simulink model "fuzzy_controller_7_trimf"  (Simulink 7.2)
settings: Solver=ode45  StartTime=0.0  StopTime=10.0  RelTol=1e-3
values from neighbouring files (symbols this model uses):
  fi_1_a = -0.786    [fuzzy_controller_3_trimf_params.m]    (also in fuzzy_controller_5_gbell_params.m = 0.1768; fuzzy_controller_5_trimf_optimal_params.m; fuzzy_controller_5_trimf_params.m; fuzzy_controller_7_trimf_params.m)
  fi_1_b = -0.786    [fuzzy_controller_3_trimf_params.m]    (also in fuzzy_controller_5_gbell_params.m = 3.278; fuzzy_controller_5_trimf_optimal_params.m; fuzzy_controller_5_trimf_params.m; fuzzy_controller_7_trimf_params.m)
  fi_1_c = 0    [fuzzy_controller_3_trimf_params.m]    (also in fuzzy_controller_5_gbell_params.m = -0.7664; fuzzy_controller_5_trimf_optimal_params.m = -0.1; fuzzy_controller_5_trimf_params.m = -0.393; fuzzy_controller_7_trimf_params.m = -0.523)
  fi_2_a = -0.786    [fuzzy_controller_3_trimf_params.m]    (also in fuzzy_controller_5_gbell_params.m = 0.1965; fuzzy_controller_5_trimf_optimal_params.m = -0.1; fuzzy_controller_5_trimf_params.m; fuzzy_controller_7_trimf_params.m)
  fi_2_b = 0    [fuzzy_controller_3_trimf_params.m]    (also in fuzzy_controller_5_gbell_params.m = 3.278; fuzzy_controller_5_trimf_optimal_params.m = -0.05; fuzzy_controller_5_trimf_params.m = -0.393; fuzzy_controller_7_trimf_params.m = -0.5238)
  fi_2_c = 0.786    [fuzzy_controller_3_trimf_params.m]    (also in fuzzy_controller_5_gbell_params.m = -0.393; fuzzy_controller_5_trimf_optimal_params.m = 0; fuzzy_controller_5_trimf_params.m = 0; fuzzy_controller_7_trimf_params.m = -0.262)
  fi_3_a = 0    [fuzzy_controller_3_trimf_params.m]    (also in fuzzy_controller_5_gbell_params.m = 0.1965; fuzzy_controller_5_trimf_optimal_params.m = -0.05; fuzzy_controller_5_trimf_params.m = -0.393; fuzzy_controller_7_trimf_params.m = -0.523)
  fi_3_b = 0.786    [fuzzy_controller_3_trimf_params.m]    (also in fuzzy_controller_5_gbell_params.m = 3.278; fuzzy_controller_5_trimf_optimal_params.m = 0; fuzzy_controller_5_trimf_params.m = 0; fuzzy_controller_7_trimf_params.m = -0.262)
  fi_3_c = 0.786    [fuzzy_controller_3_trimf_params.m]    (also in fuzzy_controller_5_gbell_params.m = 0; fuzzy_controller_5_trimf_optimal_params.m = 0.05; fuzzy_controller_5_trimf_params.m = 0.393; fuzzy_controller_7_trimf_params.m = 0)
  fi_4_a = 0.1965    [fuzzy_controller_5_gbell_params.m]    (also in fuzzy_controller_5_trimf_optimal_params.m = 0; fuzzy_controller_5_trimf_params.m = 0; fuzzy_controller_7_trimf_params.m = -0.262)
  fi_4_b = 3.278    [fuzzy_controller_5_gbell_params.m]    (also in fuzzy_controller_5_trimf_optimal_params.m = 0.05; fuzzy_controller_5_trimf_params.m = 0.393; fuzzy_controller_7_trimf_params.m = 0)
  fi_4_c = 0.393    [fuzzy_controller_5_gbell_params.m]    (also in fuzzy_controller_5_trimf_optimal_params.m = 0.1; fuzzy_controller_5_trimf_params.m = 0.786; fuzzy_controller_7_trimf_params.m = 0.262)
  fi_5_a = 0.1768    [fuzzy_controller_5_gbell_params.m]    (also in fuzzy_controller_5_trimf_optimal_params.m = 0.05; fuzzy_controller_5_trimf_params.m = 0.393; fuzzy_controller_7_trimf_params.m = 0)
  fi_5_b = 3.278    [fuzzy_controller_5_gbell_params.m]    (also in fuzzy_controller_5_trimf_optimal_params.m = 0.1; fuzzy_controller_5_trimf_params.m = 0.786; fuzzy_controller_7_trimf_params.m = 0.262)
  fi_5_c = 0.7664    [fuzzy_controller_5_gbell_params.m]    (also in fuzzy_controller_5_trimf_optimal_params.m = 0.786; fuzzy_controller_5_trimf_params.m = 0.786; fuzzy_controller_7_trimf_params.m = 0.523)
  fi_6_a = 0.262    [fuzzy_controller_7_trimf_params.m]
  fi_6_b = 0.523    [fuzzy_controller_7_trimf_params.m]
  fi_6_c = 0.786    [fuzzy_controller_7_trimf_params.m]
  fi_7_a = 0.523    [fuzzy_controller_7_trimf_params.m]
  fi_7_b = 0.786    [fuzzy_controller_7_trimf_params.m]
  fi_7_c = 0.786    [fuzzy_controller_7_trimf_params.m]
  FORCE_1_a = -150    [fuzzy_controller_3_trimf_params.m]    (also in fuzzy_controller_5_trimf_optimal_params.m; fuzzy_controller_5_trimf_params.m; fuzzy_controller_7_trimf_params.m)
  FORCE_1_b = -150    [fuzzy_controller_3_trimf_params.m]    (also in fuzzy_controller_5_trimf_optimal_params.m; fuzzy_controller_5_trimf_params.m; fuzzy_controller_7_trimf_params.m)
  FORCE_1_c = 0    [fuzzy_controller_3_trimf_params.m]    (also in fuzzy_controller_5_trimf_optimal_params.m = -75; fuzzy_controller_5_trimf_params.m = -75; fuzzy_controller_7_trimf_params.m = -100)
  FORCE_2_a = -150    [fuzzy_controller_3_trimf_params.m]    (also in fuzzy_controller_5_trimf_optimal_params.m; fuzzy_controller_5_trimf_params.m; fuzzy_controller_7_trimf_params.m)
  FORCE_2_b = 0    [fuzzy_controller_3_trimf_params.m]    (also in fuzzy_controller_5_trimf_optimal_params.m = -75; fuzzy_controller_5_trimf_params.m = -75; fuzzy_controller_7_trimf_params.m = -100)
  FORCE_2_c = 150    [fuzzy_controller_3_trimf_params.m]    (also in fuzzy_controller_5_trimf_optimal_params.m = 0; fuzzy_controller_5_trimf_params.m = 0; fuzzy_controller_7_trimf_params.m = -50)
  FORCE_3_a = 0    [fuzzy_controller_3_trimf_params.m]    (also in fuzzy_controller_5_trimf_optimal_params.m = -75; fuzzy_controller_5_trimf_params.m = -75; fuzzy_controller_7_trimf_params.m = -100)
  FORCE_3_b = 150    [fuzzy_controller_3_trimf_params.m]    (also in fuzzy_controller_5_trimf_optimal_params.m = 0; fuzzy_controller_5_trimf_params.m = 0; fuzzy_controller_7_trimf_params.m = -50)
  FORCE_3_c = 150    [fuzzy_controller_3_trimf_params.m]    (also in fuzzy_controller_5_trimf_optimal_params.m = 75; fuzzy_controller_5_trimf_params.m = 75; fuzzy_controller_7_trimf_params.m = 0)
  FORCE_4_a = 0    [fuzzy_controller_5_trimf_optimal_params.m]    (also in fuzzy_controller_5_trimf_params.m; fuzzy_controller_7_trimf_params.m = -50)
  FORCE_4_b = 75    [fuzzy_controller_5_trimf_optimal_params.m]    (also in fuzzy_controller_5_trimf_params.m; fuzzy_controller_7_trimf_params.m = 0)
  FORCE_4_c = 150    [fuzzy_controller_5_trimf_optimal_params.m]    (also in fuzzy_controller_5_trimf_params.m; fuzzy_controller_7_trimf_params.m = 50)
  FORCE_5_a = 75    [fuzzy_controller_5_trimf_optimal_params.m]    (also in fuzzy_controller_5_trimf_params.m; fuzzy_controller_7_trimf_params.m = 0)
  FORCE_5_b = 150    [fuzzy_controller_5_trimf_optimal_params.m]    (also in fuzzy_controller_5_trimf_params.m; fuzzy_controller_7_trimf_params.m = 50)
  FORCE_5_c = 150    [fuzzy_controller_5_trimf_optimal_params.m]    (also in fuzzy_controller_5_trimf_params.m; fuzzy_controller_7_trimf_params.m = 100)
  FORCE_6_a = 50    [fuzzy_controller_7_trimf_params.m]
  FORCE_6_b = 100    [fuzzy_controller_7_trimf_params.m]
  FORCE_6_c = 150    [fuzzy_controller_7_trimf_params.m]
  FORCE_7_a = 100    [fuzzy_controller_7_trimf_params.m]
  FORCE_7_b = 150    [fuzzy_controller_7_trimf_params.m]
  FORCE_7_c = 150    [fuzzy_controller_7_trimf_params.m]
  FORCE_Range_1 = -150    [fuzzy_controller_3_trimf_params.m]    (also in fuzzy_controller_5_gauss_params.m; fuzzy_controller_5_gbell_params.m; fuzzy_controller_5_trimf_optimal_params.m; fuzzy_controller_5_trimf_params.m)
  FORCE_Range_2 = 150    [fuzzy_controller_3_trimf_params.m]    (also in fuzzy_controller_5_gauss_params.m; fuzzy_controller_5_gbell_params.m; fuzzy_controller_5_trimf_optimal_params.m; fuzzy_controller_5_trimf_params.m)
  omega_1_a = -1.57    [fuzzy_controller_3_trimf_params.m]    (also in fuzzy_controller_5_gbell_params.m = 0.3532; fuzzy_controller_5_trimf_optimal_params.m; fuzzy_controller_5_trimf_params.m; fuzzy_controller_7_trimf_params.m)
  omega_1_b = -1.57    [fuzzy_controller_3_trimf_params.m]    (also in fuzzy_controller_5_gbell_params.m = 3.278; fuzzy_controller_5_trimf_optimal_params.m; fuzzy_controller_5_trimf_params.m; fuzzy_controller_7_trimf_params.m)
  omega_1_c = 0    [fuzzy_controller_3_trimf_params.m]    (also in fuzzy_controller_5_gbell_params.m = -1.531; fuzzy_controller_5_trimf_optimal_params.m = -0.86; fuzzy_controller_5_trimf_params.m = -0.785; fuzzy_controller_7_trimf_params.m = -1.047)
  omega_2_a = -1.57    [fuzzy_controller_3_trimf_params.m]    (also in fuzzy_controller_5_gbell_params.m = 0.3925; fuzzy_controller_5_trimf_optimal_params.m = -0.86; fuzzy_controller_5_trimf_params.m; fuzzy_controller_7_trimf_params.m)
  omega_2_b = 0    [fuzzy_controller_3_trimf_params.m]    (also in fuzzy_controller_5_gbell_params.m = 3.278; fuzzy_controller_5_trimf_optimal_params.m = -0.43; fuzzy_controller_5_trimf_params.m = -0.785; fuzzy_controller_7_trimf_params.m = -1.047)
  omega_2_c = 1.57    [fuzzy_controller_3_trimf_params.m]    (also in fuzzy_controller_5_gbell_params.m = -0.785; fuzzy_controller_5_trimf_optimal_params.m = 0; fuzzy_controller_5_trimf_params.m = 0; fuzzy_controller_7_trimf_params.m = -0.523)
  omega_3_a = 0    [fuzzy_controller_3_trimf_params.m]    (also in fuzzy_controller_5_gbell_params.m = 0.3925; fuzzy_controller_5_trimf_optimal_params.m = -0.43; fuzzy_controller_5_trimf_params.m = -0.785; fuzzy_controller_7_trimf_params.m = -1.047)
  omega_3_b = 1.57    [fuzzy_controller_3_trimf_params.m]    (also in fuzzy_controller_5_gbell_params.m = 3.278; fuzzy_controller_5_trimf_optimal_params.m = 0; fuzzy_controller_5_trimf_params.m = 0; fuzzy_controller_7_trimf_params.m = -0.523)
  omega_3_c = 1.57    [fuzzy_controller_3_trimf_params.m]    (also in fuzzy_controller_5_gbell_params.m = 0; fuzzy_controller_5_trimf_optimal_params.m = 0.43; fuzzy_controller_5_trimf_params.m = 0.785; fuzzy_controller_7_trimf_params.m = 0)
  omega_4_a = 0.3925    [fuzzy_controller_5_gbell_params.m]    (also in fuzzy_controller_5_trimf_optimal_params.m = 0; fuzzy_controller_5_trimf_params.m = 0; fuzzy_controller_7_trimf_params.m = -0.523)
  omega_4_b = 3.278    [fuzzy_controller_5_gbell_params.m]    (also in fuzzy_controller_5_trimf_optimal_params.m = 0.43; fuzzy_controller_5_trimf_params.m = 0.785; fuzzy_controller_7_trimf_params.m = 0)
  omega_4_c = 0.785    [fuzzy_controller_5_gbell_params.m]    (also in fuzzy_controller_5_trimf_optimal_params.m = 0.86; fuzzy_controller_5_trimf_params.m = 1.57; fuzzy_controller_7_trimf_params.m = 0.523)
  omega_5_a = 0.3532    [fuzzy_controller_5_gbell_params.m]    (also in fuzzy_controller_5_trimf_optimal_params.m = 0.43; fuzzy_controller_5_trimf_params.m = 0.785; fuzzy_controller_7_trimf_params.m = 0)
  omega_5_b = 3.278    [fuzzy_controller_5_gbell_params.m]    (also in fuzzy_controller_5_trimf_optimal_params.m = 0.86; fuzzy_controller_5_trimf_params.m = 1.57; fuzzy_controller_7_trimf_params.m = 0.523)
  omega_5_c = 1.531    [fuzzy_controller_5_gbell_params.m]    (also in fuzzy_controller_5_trimf_optimal_params.m = 1.57; fuzzy_controller_5_trimf_params.m = 1.57; fuzzy_controller_7_trimf_params.m = 1.047)
  omega_6_a = 0.523    [fuzzy_controller_7_trimf_params.m]
  omega_6_b = 1.047    [fuzzy_controller_7_trimf_params.m]
  omega_6_c = 1.57    [fuzzy_controller_7_trimf_params.m]
  omega_7_a = 1.047    [fuzzy_controller_7_trimf_params.m]
  omega_7_b = 1.57    [fuzzy_controller_7_trimf_params.m]
  omega_7_c = 1.57    [fuzzy_controller_7_trimf_params.m]
(part 2 of 4)

== system fuzzy_controller_7_trimf/Fuzzy Logic Controller/Rule39 ==
  Antecedents : Inport
  Consequents : Inport  Port=2
  Weight : Constant
  Weighting : Product  SaturateOnIntegerOverflow=on  RndMeth=Zero  InputSameDT=on  OutDataTypeStr=Inherit: Same as first input
  andorMethod : MinMax  SaturateOnIntegerOverflow=on  InputSameDT=on
  impMethod : MinMax  Inputs=2  SaturateOnIntegerOverflow=on  InputSameDT=on
  Output : Outport
  Firing Strength : Outport  Port=2
  wires:
  impMethod/1 -> Output/1
  Weighting/1 -> Firing Strength/1, impMethod/1
  Consequents/1 -> impMethod/2
  Weight/1 -> Weighting/1
  andorMethod/1 -> Weighting/2
  Antecedents/1 -> andorMethod/1

== system fuzzy_controller_7_trimf/Fuzzy Logic Controller/Rule4 ==
  Antecedents : Inport
  Consequents : Inport  Port=2
  Weight : Constant
  Weighting : Product  SaturateOnIntegerOverflow=on  RndMeth=Zero  InputSameDT=on  OutDataTypeStr=Inherit: Same as first input
  andorMethod : MinMax  SaturateOnIntegerOverflow=on  InputSameDT=on
  impMethod : MinMax  Inputs=2  SaturateOnIntegerOverflow=on  InputSameDT=on
  Output : Outport
  Firing Strength : Outport  Port=2
  wires:
  impMethod/1 -> Output/1
  Weighting/1 -> Firing Strength/1, impMethod/1
  Consequents/1 -> impMethod/2
  Weight/1 -> Weighting/1
  andorMethod/1 -> Weighting/2
  Antecedents/1 -> andorMethod/1

== system fuzzy_controller_7_trimf/Fuzzy Logic Controller/Rule40 ==
  Antecedents : Inport
  Consequents : Inport  Port=2
  Weight : Constant
  Weighting : Product  SaturateOnIntegerOverflow=on  RndMeth=Zero  InputSameDT=on  OutDataTypeStr=Inherit: Same as first input
  andorMethod : MinMax  SaturateOnIntegerOverflow=on  InputSameDT=on
  impMethod : MinMax  Inputs=2  SaturateOnIntegerOverflow=on  InputSameDT=on
  Output : Outport
  Firing Strength : Outport  Port=2
  wires:
  impMethod/1 -> Output/1
  Weighting/1 -> Firing Strength/1, impMethod/1
  Consequents/1 -> impMethod/2
  Weight/1 -> Weighting/1
  andorMethod/1 -> Weighting/2
  Antecedents/1 -> andorMethod/1

== system fuzzy_controller_7_trimf/Fuzzy Logic Controller/Rule41 ==
  Antecedents : Inport
  Consequents : Inport  Port=2
  Weight : Constant
  Weighting : Product  SaturateOnIntegerOverflow=on  RndMeth=Zero  InputSameDT=on  OutDataTypeStr=Inherit: Same as first input
  andorMethod : MinMax  SaturateOnIntegerOverflow=on  InputSameDT=on
  impMethod : MinMax  Inputs=2  SaturateOnIntegerOverflow=on  InputSameDT=on
  Output : Outport
  Firing Strength : Outport  Port=2
  wires:
  impMethod/1 -> Output/1
  Weighting/1 -> Firing Strength/1, impMethod/1
  Consequents/1 -> impMethod/2
  Weight/1 -> Weighting/1
  andorMethod/1 -> Weighting/2
  Antecedents/1 -> andorMethod/1

== system fuzzy_controller_7_trimf/Fuzzy Logic Controller/Rule42 ==
  Antecedents : Inport
  Consequents : Inport  Port=2
  Weight : Constant
  Weighting : Product  SaturateOnIntegerOverflow=on  RndMeth=Zero  InputSameDT=on  OutDataTypeStr=Inherit: Same as first input
  andorMethod : MinMax  SaturateOnIntegerOverflow=on  InputSameDT=on
  impMethod : MinMax  Inputs=2  SaturateOnIntegerOverflow=on  InputSameDT=on
  Output : Outport
  Firing Strength : Outport  Port=2
  wires:
  impMethod/1 -> Output/1
  Weighting/1 -> Firing Strength/1, impMethod/1
  Consequents/1 -> impMethod/2
  Weight/1 -> Weighting/1
  andorMethod/1 -> Weighting/2
  Antecedents/1 -> andorMethod/1

== system fuzzy_controller_7_trimf/Fuzzy Logic Controller/Rule43 ==
  Antecedents : Inport
  Consequents : Inport  Port=2
  Weight : Constant
  Weighting : Product  SaturateOnIntegerOverflow=on  RndMeth=Zero  InputSameDT=on  OutDataTypeStr=Inherit: Same as first input
  andorMethod : MinMax  SaturateOnIntegerOverflow=on  InputSameDT=on
  impMethod : MinMax  Inputs=2  SaturateOnIntegerOverflow=on  InputSameDT=on
  Output : Outport
  Firing Strength : Outport  Port=2
  wires:
  impMethod/1 -> Output/1
  Weighting/1 -> Firing Strength/1, impMethod/1
  Consequents/1 -> impMethod/2
  Weight/1 -> Weighting/1
  andorMethod/1 -> Weighting/2
  Antecedents/1 -> andorMethod/1

== system fuzzy_controller_7_trimf/Fuzzy Logic Controller/Rule44 ==
  Antecedents : Inport
  Consequents : Inport  Port=2
  Weight : Constant
  Weighting : Product  SaturateOnIntegerOverflow=on  RndMeth=Zero  InputSameDT=on  OutDataTypeStr=Inherit: Same as first input
  andorMethod : MinMax  SaturateOnIntegerOverflow=on  InputSameDT=on
  impMethod : MinMax  Inputs=2  SaturateOnIntegerOverflow=on  InputSameDT=on
  Output : Outport
  Firing Strength : Outport  Port=2
  wires:
  impMethod/1 -> Output/1
  Weighting/1 -> Firing Strength/1, impMethod/1
  Consequents/1 -> impMethod/2
  Weight/1 -> Weighting/1
  andorMethod/1 -> Weighting/2
  Antecedents/1 -> andorMethod/1

== system fuzzy_controller_7_trimf/Fuzzy Logic Controller/Rule45 ==
  Antecedents : Inport
  Consequents : Inport  Port=2
  Weight : Constant
  Weighting : Product  SaturateOnIntegerOverflow=on  RndMeth=Zero  InputSameDT=on  OutDataTypeStr=Inherit: Same as first input
  andorMethod : MinMax  SaturateOnIntegerOverflow=on  InputSameDT=on
  impMethod : MinMax  Inputs=2  SaturateOnIntegerOverflow=on  InputSameDT=on
  Output : Outport
  Firing Strength : Outport  Port=2
  wires:
  impMethod/1 -> Output/1
  Weighting/1 -> Firing Strength/1, impMethod/1
  Consequents/1 -> impMethod/2
  Weight/1 -> Weighting/1
  andorMethod/1 -> Weighting/2
  Antecedents/1 -> andorMethod/1

== system fuzzy_controller_7_trimf/Fuzzy Logic Controller/Rule46 ==
  Antecedents : Inport
  Consequents : Inport  Port=2
  Weight : Constant
  Weighting : Product  SaturateOnIntegerOverflow=on  RndMeth=Zero  InputSameDT=on  OutDataTypeStr=Inherit: Same as first input
  andorMethod : MinMax  SaturateOnIntegerOverflow=on  InputSameDT=on
  impMethod : MinMax  Inputs=2  SaturateOnIntegerOverflow=on  InputSameDT=on
  Output : Outport
  Firing Strength : Outport  Port=2
  wires:
  impMethod/1 -> Output/1
  Weighting/1 -> Firing Strength/1, impMethod/1
  Consequents/1 -> impMethod/2
  Weight/1 -> Weighting/1
  andorMethod/1 -> Weighting/2
  Antecedents/1 -> andorMethod/1

== system fuzzy_controller_7_trimf/Fuzzy Logic Controller/Rule47 ==
  Antecedents : Inport
  Consequents : Inport  Port=2
  Weight : Constant
  Weighting : Product  SaturateOnIntegerOverflow=on  RndMeth=Zero  InputSameDT=on  OutDataTypeStr=Inherit: Same as first input
  andorMethod : MinMax  SaturateOnIntegerOverflow=on  InputSameDT=on
  impMethod : MinMax  Inputs=2  SaturateOnIntegerOverflow=on  InputSameDT=on
  Output : Outport
  Firing Strength : Outport  Port=2
  wires:
  impMethod/1 -> Output/1
  Weighting/1 -> Firing Strength/1, impMethod/1
  Consequents/1 -> impMethod/2
  Weight/1 -> Weighting/1
  andorMethod/1 -> Weighting/2
  Antecedents/1 -> andorMethod/1

== system fuzzy_controller_7_trimf/Fuzzy Logic Controller/Rule48 ==
  Antecedents : Inport
  Consequents : Inport  Port=2
  Weight : Constant
  Weighting : Product  SaturateOnIntegerOverflow=on  RndMeth=Zero  InputSameDT=on  OutDataTypeStr=Inherit: Same as first input
  andorMethod : MinMax  SaturateOnIntegerOverflow=on  InputSameDT=on
  impMethod : MinMax  Inputs=2  SaturateOnIntegerOverflow=on  InputSameDT=on
  Output : Outport
  Firing Strength : Outport  Port=2
  wires:
  impMethod/1 -> Output/1
  Weighting/1 -> Firing Strength/1, impMethod/1
  Consequents/1 -> impMethod/2
  Weight/1 -> Weighting/1
  andorMethod/1 -> Weighting/2
  Antecedents/1 -> andorMethod/1

== system fuzzy_controller_7_trimf/Fuzzy Logic Controller/Rule49 ==
  Antecedents : Inport
  Consequents : Inport  Port=2
  Weight : Constant
  Weighting : Product  SaturateOnIntegerOverflow=on  RndMeth=Zero  InputSameDT=on  OutDataTypeStr=Inherit: Same as first input
  andorMethod : MinMax  SaturateOnIntegerOverflow=on  InputSameDT=on
  impMethod : MinMax  Inputs=2  SaturateOnIntegerOverflow=on  InputSameDT=on
  Output : Outport
  Firing Strength : Outport  Port=2
  wires:
  impMethod/1 -> Output/1
  Weighting/1 -> Firing Strength/1, impMethod/1
  Consequents/1 -> impMethod/2
  Weight/1 -> Weighting/1
  andorMethod/1 -> Weighting/2
  Antecedents/1 -> andorMethod/1

== system fuzzy_controller_7_trimf/Fuzzy Logic Controller/Rule5 ==
  Antecedents : Inport
  Consequents : Inport  Port=2
  Weight : Constant
  Weighting : Product  SaturateOnIntegerOverflow=on  RndMeth=Zero  InputSameDT=on  OutDataTypeStr=Inherit: Same as first input
  andorMethod : MinMax  SaturateOnIntegerOverflow=on  InputSameDT=on
  impMethod : MinMax  Inputs=2  SaturateOnIntegerOverflow=on  InputSameDT=on
  Output : Outport
  Firing Strength : Outport  Port=2
  wires:
  impMethod/1 -> Output/1
  Weighting/1 -> Firing Strength/1, impMethod/1
  Consequents/1 -> impMethod/2
  Weight/1 -> Weighting/1
  andorMethod/1 -> Weighting/2
  Antecedents/1 -> andorMethod/1

== system fuzzy_controller_7_trimf/Fuzzy Logic Controller/Rule6 ==
  Antecedents : Inport
  Consequents : Inport  Port=2
  Weight : Constant
  Weighting : Product  SaturateOnIntegerOverflow=on  RndMeth=Zero  InputSameDT=on  OutDataTypeStr=Inherit: Same as first input
  andorMethod : MinMax  SaturateOnIntegerOverflow=on  InputSameDT=on
  impMethod : MinMax  Inputs=2  SaturateOnIntegerOverflow=on  InputSameDT=on
  Output : Outport
  Firing Strength : Outport  Port=2
  wires:
  impMethod/1 -> Output/1
  Weighting/1 -> Firing Strength/1, impMethod/1
  Consequents/1 -> impMethod/2
  Weight/1 -> Weighting/1
  andorMethod/1 -> Weighting/2
  Antecedents/1 -> andorMethod/1

== system fuzzy_controller_7_trimf/Fuzzy Logic Controller/Rule7 ==
  Antecedents : Inport
  Consequents : Inport  Port=2
  Weight : Constant
  Weighting : Product  SaturateOnIntegerOverflow=on  RndMeth=Zero  InputSameDT=on  OutDataTypeStr=Inherit: Same as first input
  andorMethod : MinMax  SaturateOnIntegerOverflow=on  InputSameDT=on
  impMethod : MinMax  Inputs=2  SaturateOnIntegerOverflow=on  InputSameDT=on
  Output : Outport
  Firing Strength : Outport  Port=2
  wires:
  impMethod/1 -> Output/1
  Weighting/1 -> Firing Strength/1, impMethod/1
  Consequents/1 -> impMethod/2
  Weight/1 -> Weighting/1
  andorMethod/1 -> Weighting/2
  Antecedents/1 -> andorMethod/1

== system fuzzy_controller_7_trimf/Fuzzy Logic Controller/Rule8 ==
  Antecedents : Inport
  Consequents : Inport  Port=2
  Weight : Constant
  Weighting : Product  SaturateOnIntegerOverflow=on  RndMeth=Zero  InputSameDT=on  OutDataTypeStr=Inherit: Same as first input
  andorMethod : MinMax  SaturateOnIntegerOverflow=on  InputSameDT=on
  impMethod : MinMax  Inputs=2  SaturateOnIntegerOverflow=on  InputSameDT=on
  Output : Outport
  Firing Strength : Outport  Port=2
  wires:
  impMethod/1 -> Output/1
  Weighting/1 -> Firing Strength/1, impMethod/1
  Consequents/1 -> impMethod/2
  Weight/1 -> Weighting/1
  andorMethod/1 -> Weighting/2
  Antecedents/1 -> andorMethod/1

== system fuzzy_controller_7_trimf/Fuzzy Logic Controller/Rule9 ==
  Antecedents : Inport
  Consequents : Inport  Port=2
  Weight : Constant
  Weighting : Product  SaturateOnIntegerOverflow=on  RndMeth=Zero  InputSameDT=on  OutDataTypeStr=Inherit: Same as first input
  andorMethod : MinMax  SaturateOnIntegerOverflow=on  InputSameDT=on
  impMethod : MinMax  Inputs=2  SaturateOnIntegerOverflow=on  InputSameDT=on
  Output : Outport
  Firing Strength : Outport  Port=2
  wires:
  impMethod/1 -> Output/1
  Weighting/1 -> Firing Strength/1, impMethod/1
  Consequents/1 -> impMethod/2
  Weight/1 -> Weighting/1
  andorMethod/1 -> Weighting/2
  Antecedents/1 -> andorMethod/1

== system fuzzy_controller_7_trimf/Fuzzy Logic Controller/fi ==
  In1 : Inport
  DataConv : DataTypeConversion  OutDataTypeMode=double  OutDataTypeStr=double
  tri mf1 : Subsystem  mask{a=fi_1_a, b=fi_1_b, c=fi_1_c}
      mask prompts: a "Left base point a:"; b "Peak location b:"; c "Right base point c:"
  tri mf2 : Subsystem  mask{a=fi_2_a, b=fi_2_b, c=fi_2_c}
      mask prompts: a "Left base point a:"; b "Peak location b:"; c "Right base point c:"
  tri mf3 : Subsystem  mask{a=fi_3_a, b=fi_3_b, c=fi_3_c}
      mask prompts: a "Left base point a:"; b "Peak location b:"; c "Right base point c:"
  tri mf4 : Subsystem  mask{a=fi_4_a, b=fi_4_b, c=fi_4_c}
      mask prompts: a "Left base point a:"; b "Peak location b:"; c "Right base point c:"
  tri mf5 : Subsystem  mask{a=fi_5_a, b=fi_5_b, c=fi_5_c}
      mask prompts: a "Left base point a:"; b "Peak location b:"; c "Right base point c:"
  tri mf6 : Subsystem  mask{a=fi_6_a, b=fi_6_b, c=fi_6_c}
      mask prompts: a "Left base point a:"; b "Peak location b:"; c "Right base point c:"
  tri mf7 : Subsystem  mask{a=fi_7_a, b=fi_7_b, c=fi_7_c}
      mask prompts: a "Left base point a:"; b "Peak location b:"; c "Right base point c:"
  Out1 : Outport
  Out2 : Outport  Port=2
  Out3 : Outport  Port=3
  Out4 : Outport  Port=4
  Out5 : Outport  Port=5
  Out6 : Outport  Port=6
  Out7 : Outport  Port=7
  wires:
  In1/1 -> DataConv/1
  tri mf1/1(MF) -> Out1/1
  tri mf2/1(MF) -> Out2/1
  tri mf3/1(MF) -> Out3/1
  DataConv/1 -> tri mf1/1(x), tri mf2/1(x), tri mf6/1(x), tri mf7/1(x), tri mf5/1(x), tri mf4/1(x), tri mf3/1(x)
  tri mf4/1(MF) -> Out4/1
  tri mf5/1(MF) -> Out5/1
  tri mf6/1(MF) -> Out6/1
  tri mf7/1(MF) -> Out7/1

== system fuzzy_controller_7_trimf/Fuzzy Logic Controller/omega ==
  In1 : Inport
  DataConv : DataTypeConversion  OutDataTypeMode=double  OutDataTypeStr=double
  tri mf1 : Subsystem  mask{a=omega_1_a, b=omega_1_b, c=omega_1_c}
      mask prompts: a "Left base point a:"; b "Peak location b:"; c "Right base point c:"
  tri mf2 : Subsystem  mask{a=omega_2_a, b=omega_2_b, c=omega_2_c}
      mask prompts: a "Left base point a:"; b "Peak location b:"; c "Right base point c:"
  tri mf3 : Subsystem  mask{a=omega_3_a, b=omega_3_b, c=omega_3_c}
      mask prompts: a "Left base point a:"; b "Peak location b:"; c "Right base point c:"
  tri mf4 : Subsystem  mask{a=omega_4_a, b=omega_4_b, c=omega_4_c}
      mask prompts: a "Left base point a:"; b "Peak location b:"; c "Right base point c:"
  tri mf5 : Subsystem  mask{a=omega_5_a, b=omega_5_b, c=omega_5_c}
      mask prompts: a "Left base point a:"; b "Peak location b:"; c "Right base point c:"
  tri mf6 : Subsystem  mask{a=omega_6_a, b=omega_6_b, c=omega_6_c}
      mask prompts: a "Left base point a:"; b "Peak location b:"; c "Right base point c:"
  tri mf7 : Subsystem  mask{a=omega_7_a, b=omega_7_b, c=omega_7_c}
      mask prompts: a "Left base point a:"; b "Peak location b:"; c "Right base point c:"
  Out1 : Outport
  Out2 : Outport  Port=2
  Out3 : Outport  Port=3
  Out4 : Outport  Port=4
  Out5 : Outport  Port=5
  Out6 : Outport  Port=6
  Out7 : Outport  Port=7
  wires:
  In1/1 -> DataConv/1
  tri mf1/1(MF) -> Out1/1
  tri mf2/1(MF) -> Out2/1
  tri mf3/1(MF) -> Out3/1
  DataConv/1 -> tri mf1/1(x), tri mf2/1(x), tri mf6/1(x), tri mf7/1(x), tri mf5/1(x), tri mf4/1(x), tri mf3/1(x)
  tri mf4/1(MF) -> Out4/1
  tri mf5/1(MF) -> Out5/1
  tri mf6/1(MF) -> Out6/1
  tri mf7/1(MF) -> Out7/1

== system fuzzy_controller_7_trimf/Fuzzy Logic Controller/Defuzzification/Action: One ==
  Action Port : ActionPort
  One : Constant
  Out1 : Outport  InitialOutput=0
  wires:
  One/1 -> Out1/1

== system fuzzy_controller_7_trimf/Fuzzy Logic Controller/Defuzzification/Action: u1 ==
  u1 : Inport  SampleTime=[0 1]
  Action Port : ActionPort
  u2 : Outport  InitialOutput=0
  wires:
  u1/1 -> u2/1

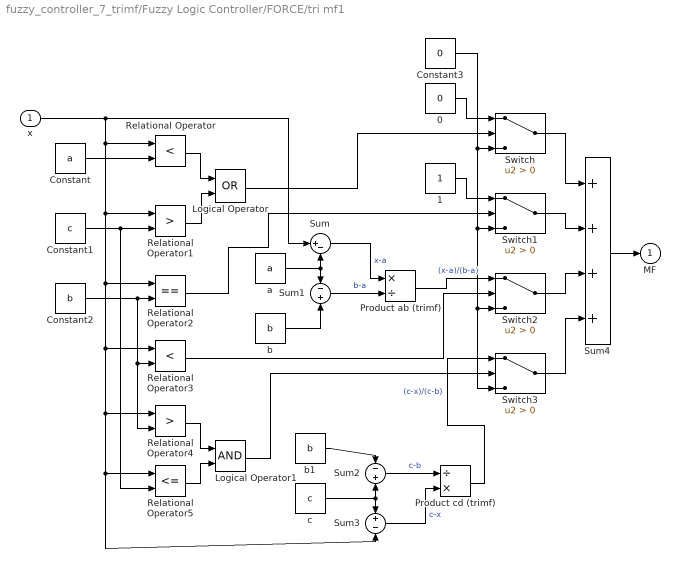
== system fuzzy_controller_7_trimf/Fuzzy Logic Controller/FORCE/tri mf1 ==
  x : Inport
  0 : Constant  Value=0
  1 : Constant
  Constant : Constant  Value=a
  Constant1 : Constant  Value=c
  Constant2 : Constant  Value=b
  Constant3 : Constant  Value=0
  Logical Operator : Logic  Operator=OR  AllPortsSameDT=off  OutDataTypeMode=boolean  OutDataTypeStr=boolean
  Logical Operator1 : Logic  AllPortsSameDT=off  OutDataTypeMode=boolean  OutDataTypeStr=boolean
  Product ab (trimf) : Product  Inputs=*/  SaturateOnIntegerOverflow=on  InputSameDT=on  OutDataTypeStr=Inherit: Same as first input
  Product cd (trimf) : Product  Inputs=/*  SaturateOnIntegerOverflow=on  InputSameDT=on  OutDataTypeStr=Inherit: Same as first input
  Relational Operator : RelationalOperator  Operator=<  LogicOutDataTypeMode=boolean  OutDataTypeStr=boolean
  Relational Operator1 : RelationalOperator  Operator=>  LogicOutDataTypeMode=boolean  OutDataTypeStr=boolean
  Relational Operator2 : RelationalOperator  Operator===  LogicOutDataTypeMode=boolean  OutDataTypeStr=boolean
  Relational Operator3 : RelationalOperator  Operator=<  LogicOutDataTypeMode=boolean  OutDataTypeStr=boolean
  Relational Operator4 : RelationalOperator  Operator=>  LogicOutDataTypeMode=boolean  OutDataTypeStr=boolean
  Relational Operator5 : RelationalOperator  Operator=<=  LogicOutDataTypeMode=boolean  OutDataTypeStr=boolean
  Sum : Sum  Inputs=|+-  SaturateOnIntegerOverflow=on  InputSameDT=on  OutDataTypeStr=Inherit: Same as first input
  Sum1 : Sum  Inputs=-+  SaturateOnIntegerOverflow=on  InputSameDT=on  OutDataTypeStr=Inherit: Same as first input
  Sum2 : Sum  Inputs=-+  SaturateOnIntegerOverflow=on  InputSameDT=on  OutDataTypeStr=Inherit: Same as first input
  Sum3 : Sum  Inputs=+-  SaturateOnIntegerOverflow=on  InputSameDT=on  OutDataTypeStr=Inherit: Same as first input
  Sum4 : Sum  Inputs=++++
  Switch{,1..3} (4 alike) : Switch  Criteria=u2 > Threshold
  a : Constant  Value=a
  b : Constant  Value=b
  b1 : Constant  Value=b
  c : Constant  Value=c
  MF : Outport
  wires:
  0/1 -> Switch/1
  1/1 -> Switch1/1
  Constant/1 -> Relational Operator/2
  Relational Operator/1 -> Logical Operator/1
  Constant1/1 -> Relational Operator5/2, Relational Operator1/2
  Relational Operator1/1 -> Logical Operator/2
  Product ab (trimf)/1 -> Switch2/1  "(x-a)/(b-a)"
  a/1 -> Sum/2, Sum1/1
  b/1 -> Sum1/2
  Sum/1 -> Product ab (trimf)/1  "x-a"
  Sum1/1 -> Product ab (trimf)/2  "b-a"
  b1/1 -> Sum2/1
  x/1 -> Sum/1, Sum3/2, Relational Operator5/1, Relational Operator4/1, Relational Operator3/1, Relational Operator2/1, Relational Operator1/1, Relational Operator/1
  c/1 -> Sum3/1, Sum2/2
  Sum3/1 -> Product cd (trimf)/2  "c-x"
  Sum2/1 -> Product cd (trimf)/1  "c-b"
  Product cd (trimf)/1 -> Switch3/1  "(c-x)/(c-b)"
  Constant2/1 -> Relational Operator2/2, Relational Operator3/2, Relational Operator4/2
  Relational Operator4/1 -> Logical Operator1/1
  Relational Operator5/1 -> Logical Operator1/2
  Switch/1 -> Sum4/1
  Switch1/1 -> Sum4/2
  Switch2/1 -> Sum4/3
  Switch3/1 -> Sum4/4
  Constant3/1 -> Switch3/3, Switch2/3, Switch1/3, Switch/3
  Logical Operator1/1 -> Switch3/2
  Relational Operator3/1 -> Switch2/2
  Relational Operator2/1 -> Switch1/2
  Logical Operator/1 -> Switch/2
  Sum4/1 -> MF/1

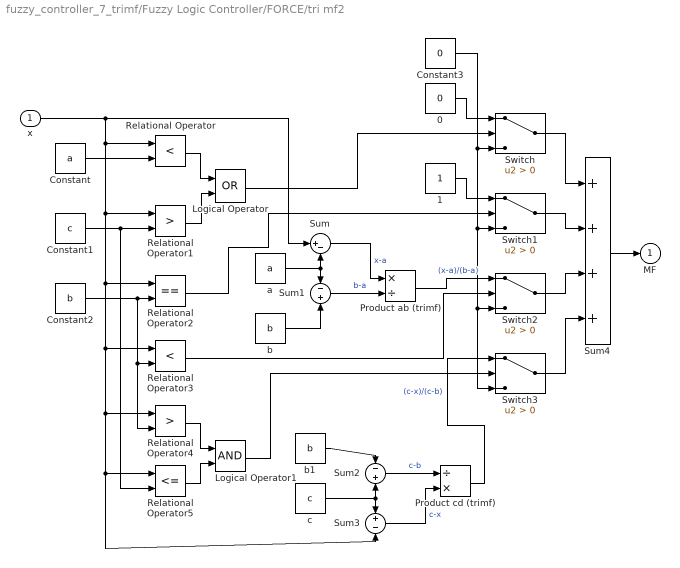
== system fuzzy_controller_7_trimf/Fuzzy Logic Controller/FORCE/tri mf2 ==
  x : Inport
  0 : Constant  Value=0
  1 : Constant
  Constant : Constant  Value=a
  Constant1 : Constant  Value=c
  Constant2 : Constant  Value=b
  Constant3 : Constant  Value=0
  Logical Operator : Logic  Operator=OR  AllPortsSameDT=off  OutDataTypeMode=boolean  OutDataTypeStr=boolean
  Logical Operator1 : Logic  AllPortsSameDT=off  OutDataTypeMode=boolean  OutDataTypeStr=boolean
  Product ab (trimf) : Product  Inputs=*/  SaturateOnIntegerOverflow=on  InputSameDT=on  OutDataTypeStr=Inherit: Same as first input
  Product cd (trimf) : Product  Inputs=/*  SaturateOnIntegerOverflow=on  InputSameDT=on  OutDataTypeStr=Inherit: Same as first input
  Relational Operator : RelationalOperator  Operator=<  LogicOutDataTypeMode=boolean  OutDataTypeStr=boolean
  Relational Operator1 : RelationalOperator  Operator=>  LogicOutDataTypeMode=boolean  OutDataTypeStr=boolean
  Relational Operator2 : RelationalOperator  Operator===  LogicOutDataTypeMode=boolean  OutDataTypeStr=boolean
  Relational Operator3 : RelationalOperator  Operator=<  LogicOutDataTypeMode=boolean  OutDataTypeStr=boolean
  Relational Operator4 : RelationalOperator  Operator=>  LogicOutDataTypeMode=boolean  OutDataTypeStr=boolean
  Relational Operator5 : RelationalOperator  Operator=<=  LogicOutDataTypeMode=boolean  OutDataTypeStr=boolean
  Sum : Sum  Inputs=|+-  SaturateOnIntegerOverflow=on  InputSameDT=on  OutDataTypeStr=Inherit: Same as first input
  Sum1 : Sum  Inputs=-+  SaturateOnIntegerOverflow=on  InputSameDT=on  OutDataTypeStr=Inherit: Same as first input
  Sum2 : Sum  Inputs=-+  SaturateOnIntegerOverflow=on  InputSameDT=on  OutDataTypeStr=Inherit: Same as first input
  Sum3 : Sum  Inputs=+-  SaturateOnIntegerOverflow=on  InputSameDT=on  OutDataTypeStr=Inherit: Same as first input
  Sum4 : Sum  Inputs=++++
  Switch{,1..3} (4 alike) : Switch  Criteria=u2 > Threshold
  a : Constant  Value=a
  b : Constant  Value=b
  b1 : Constant  Value=b
  c : Constant  Value=c
  MF : Outport
  wires:
  0/1 -> Switch/1
  1/1 -> Switch1/1
  Constant/1 -> Relational Operator/2
  Relational Operator/1 -> Logical Operator/1
  Constant1/1 -> Relational Operator5/2, Relational Operator1/2
  Relational Operator1/1 -> Logical Operator/2
  Product ab (trimf)/1 -> Switch2/1  "(x-a)/(b-a)"
  a/1 -> Sum/2, Sum1/1
  b/1 -> Sum1/2
  Sum/1 -> Product ab (trimf)/1  "x-a"
  Sum1/1 -> Product ab (trimf)/2  "b-a"
  b1/1 -> Sum2/1
  x/1 -> Sum/1, Sum3/2, Relational Operator5/1, Relational Operator4/1, Relational Operator3/1, Relational Operator2/1, Relational Operator1/1, Relational Operator/1
  c/1 -> Sum3/1, Sum2/2
  Sum3/1 -> Product cd (trimf)/2  "c-x"
  Sum2/1 -> Product cd (trimf)/1  "c-b"
  Product cd (trimf)/1 -> Switch3/1  "(c-x)/(c-b)"
  Constant2/1 -> Relational Operator2/2, Relational Operator3/2, Relational Operator4/2
  Relational Operator4/1 -> Logical Operator1/1
  Relational Operator5/1 -> Logical Operator1/2
  Switch/1 -> Sum4/1
  Switch1/1 -> Sum4/2
  Switch2/1 -> Sum4/3
  Switch3/1 -> Sum4/4
  Constant3/1 -> Switch3/3, Switch2/3, Switch1/3, Switch/3
  Logical Operator1/1 -> Switch3/2
  Relational Operator3/1 -> Switch2/2
  Relational Operator2/1 -> Switch1/2
  Logical Operator/1 -> Switch/2
  Sum4/1 -> MF/1

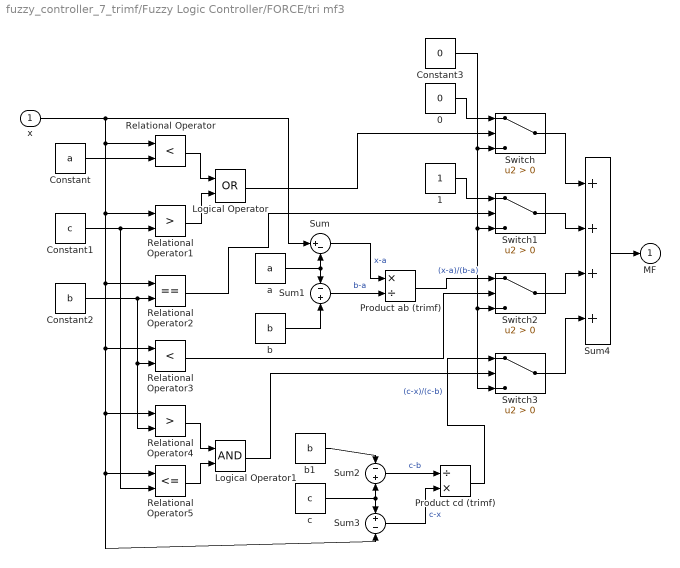
== system fuzzy_controller_7_trimf/Fuzzy Logic Controller/FORCE/tri mf3 ==
  x : Inport
  0 : Constant  Value=0
  1 : Constant
  Constant : Constant  Value=a
  Constant1 : Constant  Value=c
  Constant2 : Constant  Value=b
  Constant3 : Constant  Value=0
  Logical Operator : Logic  Operator=OR  AllPortsSameDT=off  OutDataTypeMode=boolean  OutDataTypeStr=boolean
  Logical Operator1 : Logic  AllPortsSameDT=off  OutDataTypeMode=boolean  OutDataTypeStr=boolean
  Product ab (trimf) : Product  Inputs=*/  SaturateOnIntegerOverflow=on  InputSameDT=on  OutDataTypeStr=Inherit: Same as first input
  Product cd (trimf) : Product  Inputs=/*  SaturateOnIntegerOverflow=on  InputSameDT=on  OutDataTypeStr=Inherit: Same as first input
  Relational Operator : RelationalOperator  Operator=<  LogicOutDataTypeMode=boolean  OutDataTypeStr=boolean
  Relational Operator1 : RelationalOperator  Operator=>  LogicOutDataTypeMode=boolean  OutDataTypeStr=boolean
  Relational Operator2 : RelationalOperator  Operator===  LogicOutDataTypeMode=boolean  OutDataTypeStr=boolean
  Relational Operator3 : RelationalOperator  Operator=<  LogicOutDataTypeMode=boolean  OutDataTypeStr=boolean
  Relational Operator4 : RelationalOperator  Operator=>  LogicOutDataTypeMode=boolean  OutDataTypeStr=boolean
  Relational Operator5 : RelationalOperator  Operator=<=  LogicOutDataTypeMode=boolean  OutDataTypeStr=boolean
  Sum : Sum  Inputs=|+-  SaturateOnIntegerOverflow=on  InputSameDT=on  OutDataTypeStr=Inherit: Same as first input
  Sum1 : Sum  Inputs=-+  SaturateOnIntegerOverflow=on  InputSameDT=on  OutDataTypeStr=Inherit: Same as first input
  Sum2 : Sum  Inputs=-+  SaturateOnIntegerOverflow=on  InputSameDT=on  OutDataTypeStr=Inherit: Same as first input
  Sum3 : Sum  Inputs=+-  SaturateOnIntegerOverflow=on  InputSameDT=on  OutDataTypeStr=Inherit: Same as first input
  Sum4 : Sum  Inputs=++++
  Switch{,1..3} (4 alike) : Switch  Criteria=u2 > Threshold
  a : Constant  Value=a
  b : Constant  Value=b
  b1 : Constant  Value=b
  c : Constant  Value=c
  MF : Outport
  wires:
  0/1 -> Switch/1
  1/1 -> Switch1/1
  Constant/1 -> Relational Operator/2
  Relational Operator/1 -> Logical Operator/1
  Constant1/1 -> Relational Operator5/2, Relational Operator1/2
  Relational Operator1/1 -> Logical Operator/2
  Product ab (trimf)/1 -> Switch2/1  "(x-a)/(b-a)"
  a/1 -> Sum/2, Sum1/1
  b/1 -> Sum1/2
  Sum/1 -> Product ab (trimf)/1  "x-a"
  Sum1/1 -> Product ab (trimf)/2  "b-a"
  b1/1 -> Sum2/1
  x/1 -> Sum/1, Sum3/2, Relational Operator5/1, Relational Operator4/1, Relational Operator3/1, Relational Operator2/1, Relational Operator1/1, Relational Operator/1
  c/1 -> Sum3/1, Sum2/2
  Sum3/1 -> Product cd (trimf)/2  "c-x"
  Sum2/1 -> Product cd (trimf)/1  "c-b"
  Product cd (trimf)/1 -> Switch3/1  "(c-x)/(c-b)"
  Constant2/1 -> Relational Operator2/2, Relational Operator3/2, Relational Operator4/2
  Relational Operator4/1 -> Logical Operator1/1
  Relational Operator5/1 -> Logical Operator1/2
  Switch/1 -> Sum4/1
  Switch1/1 -> Sum4/2
  Switch2/1 -> Sum4/3
  Switch3/1 -> Sum4/4
  Constant3/1 -> Switch3/3, Switch2/3, Switch1/3, Switch/3
  Logical Operator1/1 -> Switch3/2
  Relational Operator3/1 -> Switch2/2
  Relational Operator2/1 -> Switch1/2
  Logical Operator/1 -> Switch/2
  Sum4/1 -> MF/1

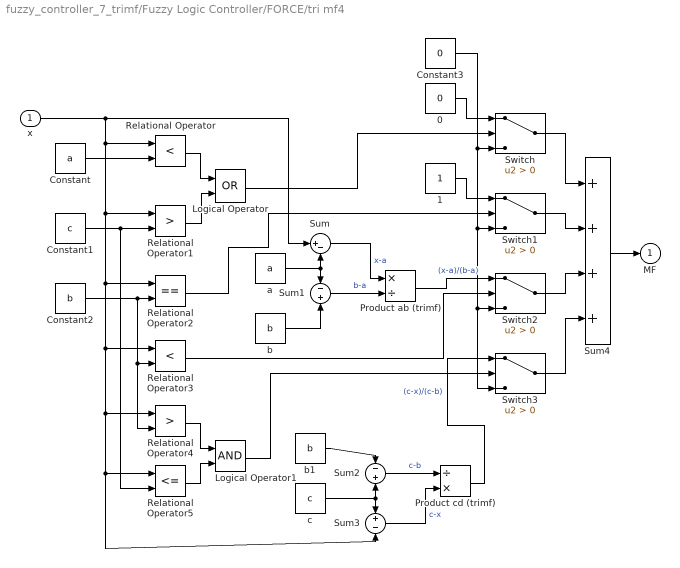
== system fuzzy_controller_7_trimf/Fuzzy Logic Controller/FORCE/tri mf4 ==
  x : Inport
  0 : Constant  Value=0
  1 : Constant
  Constant : Constant  Value=a
  Constant1 : Constant  Value=c
  Constant2 : Constant  Value=b
  Constant3 : Constant  Value=0
  Logical Operator : Logic  Operator=OR  AllPortsSameDT=off  OutDataTypeMode=boolean  OutDataTypeStr=boolean
  Logical Operator1 : Logic  AllPortsSameDT=off  OutDataTypeMode=boolean  OutDataTypeStr=boolean
  Product ab (trimf) : Product  Inputs=*/  SaturateOnIntegerOverflow=on  InputSameDT=on  OutDataTypeStr=Inherit: Same as first input
  Product cd (trimf) : Product  Inputs=/*  SaturateOnIntegerOverflow=on  InputSameDT=on  OutDataTypeStr=Inherit: Same as first input
  Relational Operator : RelationalOperator  Operator=<  LogicOutDataTypeMode=boolean  OutDataTypeStr=boolean
  Relational Operator1 : RelationalOperator  Operator=>  LogicOutDataTypeMode=boolean  OutDataTypeStr=boolean
  Relational Operator2 : RelationalOperator  Operator===  LogicOutDataTypeMode=boolean  OutDataTypeStr=boolean
  Relational Operator3 : RelationalOperator  Operator=<  LogicOutDataTypeMode=boolean  OutDataTypeStr=boolean
  Relational Operator4 : RelationalOperator  Operator=>  LogicOutDataTypeMode=boolean  OutDataTypeStr=boolean
  Relational Operator5 : RelationalOperator  Operator=<=  LogicOutDataTypeMode=boolean  OutDataTypeStr=boolean
  Sum : Sum  Inputs=|+-  SaturateOnIntegerOverflow=on  InputSameDT=on  OutDataTypeStr=Inherit: Same as first input
  Sum1 : Sum  Inputs=-+  SaturateOnIntegerOverflow=on  InputSameDT=on  OutDataTypeStr=Inherit: Same as first input
  Sum2 : Sum  Inputs=-+  SaturateOnIntegerOverflow=on  InputSameDT=on  OutDataTypeStr=Inherit: Same as first input
  Sum3 : Sum  Inputs=+-  SaturateOnIntegerOverflow=on  InputSameDT=on  OutDataTypeStr=Inherit: Same as first input
  Sum4 : Sum  Inputs=++++
  Switch{,1..3} (4 alike) : Switch  Criteria=u2 > Threshold
  a : Constant  Value=a
  b : Constant  Value=b
  b1 : Constant  Value=b
  c : Constant  Value=c
  MF : Outport
  wires:
  0/1 -> Switch/1
  1/1 -> Switch1/1
  Constant/1 -> Relational Operator/2
  Relational Operator/1 -> Logical Operator/1
  Constant1/1 -> Relational Operator5/2, Relational Operator1/2
  Relational Operator1/1 -> Logical Operator/2
  Product ab (trimf)/1 -> Switch2/1  "(x-a)/(b-a)"
  a/1 -> Sum/2, Sum1/1
  b/1 -> Sum1/2
  Sum/1 -> Product ab (trimf)/1  "x-a"
  Sum1/1 -> Product ab (trimf)/2  "b-a"
  b1/1 -> Sum2/1
  x/1 -> Sum/1, Sum3/2, Relational Operator5/1, Relational Operator4/1, Relational Operator3/1, Relational Operator2/1, Relational Operator1/1, Relational Operator/1
  c/1 -> Sum3/1, Sum2/2
  Sum3/1 -> Product cd (trimf)/2  "c-x"
  Sum2/1 -> Product cd (trimf)/1  "c-b"
  Product cd (trimf)/1 -> Switch3/1  "(c-x)/(c-b)"
  Constant2/1 -> Relational Operator2/2, Relational Operator3/2, Relational Operator4/2
  Relational Operator4/1 -> Logical Operator1/1
  Relational Operator5/1 -> Logical Operator1/2
  Switch/1 -> Sum4/1
  Switch1/1 -> Sum4/2
  Switch2/1 -> Sum4/3
  Switch3/1 -> Sum4/4
  Constant3/1 -> Switch3/3, Switch2/3, Switch1/3, Switch/3
  Logical Operator1/1 -> Switch3/2
  Relational Operator3/1 -> Switch2/2
  Relational Operator2/1 -> Switch1/2
  Logical Operator/1 -> Switch/2
  Sum4/1 -> MF/1

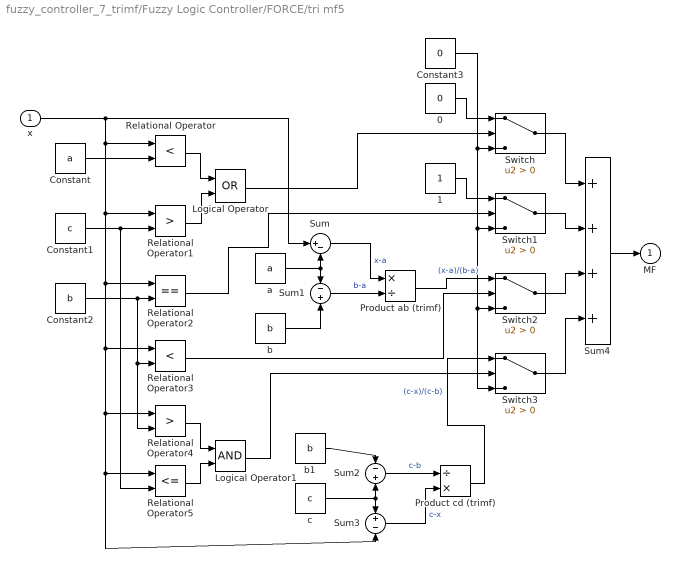
== system fuzzy_controller_7_trimf/Fuzzy Logic Controller/FORCE/tri mf5 ==
  x : Inport
  0 : Constant  Value=0
  1 : Constant
  Constant : Constant  Value=a
  Constant1 : Constant  Value=c
  Constant2 : Constant  Value=b
  Constant3 : Constant  Value=0
  Logical Operator : Logic  Operator=OR  AllPortsSameDT=off  OutDataTypeMode=boolean  OutDataTypeStr=boolean
  Logical Operator1 : Logic  AllPortsSameDT=off  OutDataTypeMode=boolean  OutDataTypeStr=boolean
  Product ab (trimf) : Product  Inputs=*/  SaturateOnIntegerOverflow=on  InputSameDT=on  OutDataTypeStr=Inherit: Same as first input
  Product cd (trimf) : Product  Inputs=/*  SaturateOnIntegerOverflow=on  InputSameDT=on  OutDataTypeStr=Inherit: Same as first input
  Relational Operator : RelationalOperator  Operator=<  LogicOutDataTypeMode=boolean  OutDataTypeStr=boolean
  Relational Operator1 : RelationalOperator  Operator=>  LogicOutDataTypeMode=boolean  OutDataTypeStr=boolean
  Relational Operator2 : RelationalOperator  Operator===  LogicOutDataTypeMode=boolean  OutDataTypeStr=boolean
  Relational Operator3 : RelationalOperator  Operator=<  LogicOutDataTypeMode=boolean  OutDataTypeStr=boolean
  Relational Operator4 : RelationalOperator  Operator=>  LogicOutDataTypeMode=boolean  OutDataTypeStr=boolean
  Relational Operator5 : RelationalOperator  Operator=<=  LogicOutDataTypeMode=boolean  OutDataTypeStr=boolean
  Sum : Sum  Inputs=|+-  SaturateOnIntegerOverflow=on  InputSameDT=on  OutDataTypeStr=Inherit: Same as first input
  Sum1 : Sum  Inputs=-+  SaturateOnIntegerOverflow=on  InputSameDT=on  OutDataTypeStr=Inherit: Same as first input
  Sum2 : Sum  Inputs=-+  SaturateOnIntegerOverflow=on  InputSameDT=on  OutDataTypeStr=Inherit: Same as first input
  Sum3 : Sum  Inputs=+-  SaturateOnIntegerOverflow=on  InputSameDT=on  OutDataTypeStr=Inherit: Same as first input
  Sum4 : Sum  Inputs=++++
  Switch{,1..3} (4 alike) : Switch  Criteria=u2 > Threshold
  a : Constant  Value=a
  b : Constant  Value=b
  b1 : Constant  Value=b
  c : Constant  Value=c
  MF : Outport
  wires:
  0/1 -> Switch/1
  1/1 -> Switch1/1
  Constant/1 -> Relational Operator/2
  Relational Operator/1 -> Logical Operator/1
  Constant1/1 -> Relational Operator5/2, Relational Operator1/2
  Relational Operator1/1 -> Logical Operator/2
  Product ab (trimf)/1 -> Switch2/1  "(x-a)/(b-a)"
  a/1 -> Sum/2, Sum1/1
  b/1 -> Sum1/2
  Sum/1 -> Product ab (trimf)/1  "x-a"
  Sum1/1 -> Product ab (trimf)/2  "b-a"
  b1/1 -> Sum2/1
  x/1 -> Sum/1, Sum3/2, Relational Operator5/1, Relational Operator4/1, Relational Operator3/1, Relational Operator2/1, Relational Operator1/1, Relational Operator/1
  c/1 -> Sum3/1, Sum2/2
  Sum3/1 -> Product cd (trimf)/2  "c-x"
  Sum2/1 -> Product cd (trimf)/1  "c-b"
  Product cd (trimf)/1 -> Switch3/1  "(c-x)/(c-b)"
  Constant2/1 -> Relational Operator2/2, Relational Operator3/2, Relational Operator4/2
  Relational Operator4/1 -> Logical Operator1/1
  Relational Operator5/1 -> Logical Operator1/2
  Switch/1 -> Sum4/1
  Switch1/1 -> Sum4/2
  Switch2/1 -> Sum4/3
  Switch3/1 -> Sum4/4
  Constant3/1 -> Switch3/3, Switch2/3, Switch1/3, Switch/3
  Logical Operator1/1 -> Switch3/2
  Relational Operator3/1 -> Switch2/2
  Relational Operator2/1 -> Switch1/2
  Logical Operator/1 -> Switch/2
  Sum4/1 -> MF/1

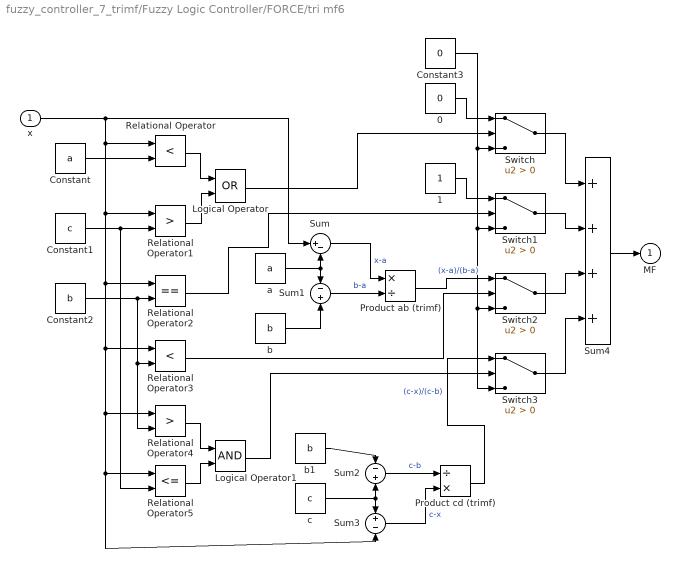
== system fuzzy_controller_7_trimf/Fuzzy Logic Controller/FORCE/tri mf6 ==
  x : Inport
  0 : Constant  Value=0
  1 : Constant
  Constant : Constant  Value=a
  Constant1 : Constant  Value=c
  Constant2 : Constant  Value=b
  Constant3 : Constant  Value=0
  Logical Operator : Logic  Operator=OR  AllPortsSameDT=off  OutDataTypeMode=boolean  OutDataTypeStr=boolean
  Logical Operator1 : Logic  AllPortsSameDT=off  OutDataTypeMode=boolean  OutDataTypeStr=boolean
  Product ab (trimf) : Product  Inputs=*/  SaturateOnIntegerOverflow=on  InputSameDT=on  OutDataTypeStr=Inherit: Same as first input
  Product cd (trimf) : Product  Inputs=/*  SaturateOnIntegerOverflow=on  InputSameDT=on  OutDataTypeStr=Inherit: Same as first input
  Relational Operator : RelationalOperator  Operator=<  LogicOutDataTypeMode=boolean  OutDataTypeStr=boolean
  Relational Operator1 : RelationalOperator  Operator=>  LogicOutDataTypeMode=boolean  OutDataTypeStr=boolean
  Relational Operator2 : RelationalOperator  Operator===  LogicOutDataTypeMode=boolean  OutDataTypeStr=boolean
  Relational Operator3 : RelationalOperator  Operator=<  LogicOutDataTypeMode=boolean  OutDataTypeStr=boolean
  Relational Operator4 : RelationalOperator  Operator=>  LogicOutDataTypeMode=boolean  OutDataTypeStr=boolean
  Relational Operator5 : RelationalOperator  Operator=<=  LogicOutDataTypeMode=boolean  OutDataTypeStr=boolean
  Sum : Sum  Inputs=|+-  SaturateOnIntegerOverflow=on  InputSameDT=on  OutDataTypeStr=Inherit: Same as first input
  Sum1 : Sum  Inputs=-+  SaturateOnIntegerOverflow=on  InputSameDT=on  OutDataTypeStr=Inherit: Same as first input
  Sum2 : Sum  Inputs=-+  SaturateOnIntegerOverflow=on  InputSameDT=on  OutDataTypeStr=Inherit: Same as first input
  Sum3 : Sum  Inputs=+-  SaturateOnIntegerOverflow=on  InputSameDT=on  OutDataTypeStr=Inherit: Same as first input
  Sum4 : Sum  Inputs=++++
  Switch{,1..3} (4 alike) : Switch  Criteria=u2 > Threshold
  a : Constant  Value=a
  b : Constant  Value=b
  b1 : Constant  Value=b
  c : Constant  Value=c
  MF : Outport
  wires:
  0/1 -> Switch/1
  1/1 -> Switch1/1
  Constant/1 -> Relational Operator/2
  Relational Operator/1 -> Logical Operator/1
  Constant1/1 -> Relational Operator5/2, Relational Operator1/2
  Relational Operator1/1 -> Logical Operator/2
  Product ab (trimf)/1 -> Switch2/1  "(x-a)/(b-a)"
  a/1 -> Sum/2, Sum1/1
  b/1 -> Sum1/2
  Sum/1 -> Product ab (trimf)/1  "x-a"
  Sum1/1 -> Product ab (trimf)/2  "b-a"
  b1/1 -> Sum2/1
  x/1 -> Sum/1, Sum3/2, Relational Operator5/1, Relational Operator4/1, Relational Operator3/1, Relational Operator2/1, Relational Operator1/1, Relational Operator/1
  c/1 -> Sum3/1, Sum2/2
  Sum3/1 -> Product cd (trimf)/2  "c-x"
  Sum2/1 -> Product cd (trimf)/1  "c-b"
  Product cd (trimf)/1 -> Switch3/1  "(c-x)/(c-b)"
  Constant2/1 -> Relational Operator2/2, Relational Operator3/2, Relational Operator4/2
  Relational Operator4/1 -> Logical Operator1/1
  Relational Operator5/1 -> Logical Operator1/2
  Switch/1 -> Sum4/1
  Switch1/1 -> Sum4/2
  Switch2/1 -> Sum4/3
  Switch3/1 -> Sum4/4
  Constant3/1 -> Switch3/3, Switch2/3, Switch1/3, Switch/3
  Logical Operator1/1 -> Switch3/2
  Relational Operator3/1 -> Switch2/2
  Relational Operator2/1 -> Switch1/2
  Logical Operator/1 -> Switch/2
  Sum4/1 -> MF/1

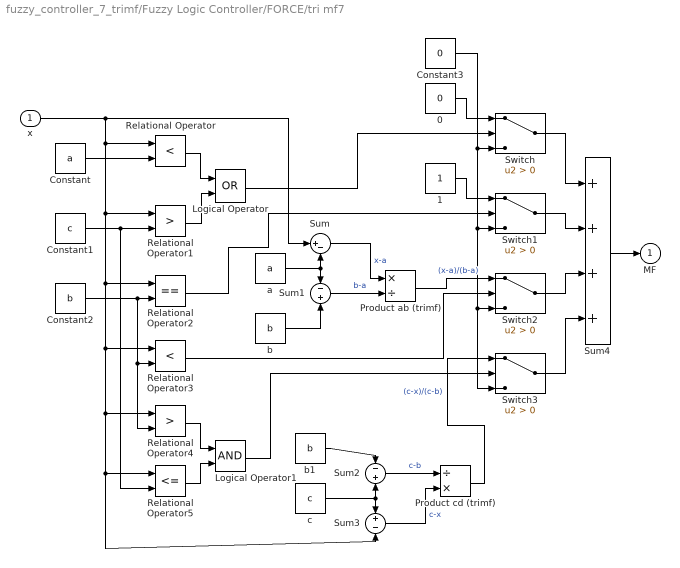
== system fuzzy_controller_7_trimf/Fuzzy Logic Controller/FORCE/tri mf7 ==
  x : Inport
  0 : Constant  Value=0
  1 : Constant
  Constant : Constant  Value=a
  Constant1 : Constant  Value=c
  Constant2 : Constant  Value=b
  Constant3 : Constant  Value=0
  Logical Operator : Logic  Operator=OR  AllPortsSameDT=off  OutDataTypeMode=boolean  OutDataTypeStr=boolean
  Logical Operator1 : Logic  AllPortsSameDT=off  OutDataTypeMode=boolean  OutDataTypeStr=boolean
  Product ab (trimf) : Product  Inputs=*/  SaturateOnIntegerOverflow=on  InputSameDT=on  OutDataTypeStr=Inherit: Same as first input
  Product cd (trimf) : Product  Inputs=/*  SaturateOnIntegerOverflow=on  InputSameDT=on  OutDataTypeStr=Inherit: Same as first input
  Relational Operator : RelationalOperator  Operator=<  LogicOutDataTypeMode=boolean  OutDataTypeStr=boolean
  Relational Operator1 : RelationalOperator  Operator=>  LogicOutDataTypeMode=boolean  OutDataTypeStr=boolean
  Relational Operator2 : RelationalOperator  Operator===  LogicOutDataTypeMode=boolean  OutDataTypeStr=boolean
  Relational Operator3 : RelationalOperator  Operator=<  LogicOutDataTypeMode=boolean  OutDataTypeStr=boolean
  Relational Operator4 : RelationalOperator  Operator=>  LogicOutDataTypeMode=boolean  OutDataTypeStr=boolean
  Relational Operator5 : RelationalOperator  Operator=<=  LogicOutDataTypeMode=boolean  OutDataTypeStr=boolean
  Sum : Sum  Inputs=|+-  SaturateOnIntegerOverflow=on  InputSameDT=on  OutDataTypeStr=Inherit: Same as first input
  Sum1 : Sum  Inputs=-+  SaturateOnIntegerOverflow=on  InputSameDT=on  OutDataTypeStr=Inherit: Same as first input
  Sum2 : Sum  Inputs=-+  SaturateOnIntegerOverflow=on  InputSameDT=on  OutDataTypeStr=Inherit: Same as first input
  Sum3 : Sum  Inputs=+-  SaturateOnIntegerOverflow=on  InputSameDT=on  OutDataTypeStr=Inherit: Same as first input
  Sum4 : Sum  Inputs=++++
  Switch{,1..3} (4 alike) : Switch  Criteria=u2 > Threshold
  a : Constant  Value=a
  b : Constant  Value=b
  b1 : Constant  Value=b
  c : Constant  Value=c
  MF : Outport
  wires:
  0/1 -> Switch/1
  1/1 -> Switch1/1
  Constant/1 -> Relational Operator/2
  Relational Operator/1 -> Logical Operator/1
  Constant1/1 -> Relational Operator5/2, Relational Operator1/2
  Relational Operator1/1 -> Logical Operator/2
  Product ab (trimf)/1 -> Switch2/1  "(x-a)/(b-a)"
  a/1 -> Sum/2, Sum1/1
  b/1 -> Sum1/2
  Sum/1 -> Product ab (trimf)/1  "x-a"
  Sum1/1 -> Product ab (trimf)/2  "b-a"
  b1/1 -> Sum2/1
  x/1 -> Sum/1, Sum3/2, Relational Operator5/1, Relational Operator4/1, Relational Operator3/1, Relational Operator2/1, Relational Operator1/1, Relational Operator/1
  c/1 -> Sum3/1, Sum2/2
  Sum3/1 -> Product cd (trimf)/2  "c-x"
  Sum2/1 -> Product cd (trimf)/1  "c-b"
  Product cd (trimf)/1 -> Switch3/1  "(c-x)/(c-b)"
  Constant2/1 -> Relational Operator2/2, Relational Operator3/2, Relational Operator4/2
  Relational Operator4/1 -> Logical Operator1/1
  Relational Operator5/1 -> Logical Operator1/2
  Switch/1 -> Sum4/1
  Switch1/1 -> Sum4/2
  Switch2/1 -> Sum4/3
  Switch3/1 -> Sum4/4
  Constant3/1 -> Switch3/3, Switch2/3, Switch1/3, Switch/3
  Logical Operator1/1 -> Switch3/2
  Relational Operator3/1 -> Switch2/2
  Relational Operator2/1 -> Switch1/2
  Logical Operator/1 -> Switch/2
  Sum4/1 -> MF/1
